simulink model "dc_motor_model_basic_blocks_current_feedback"  (Simulink 7.8)
settings: Solver=ode45  StartTime=0.0  StopTime=10.0  RelTol=1e-3
values from neighbouring files (symbols this model uses):
  I_d = 0    [dc_motor_basic_blocks_current_feedback.m]    (also in dc_motor_h_bridge_current_feedback.m)
  J = 8.85*10^(-7)    (= 8.85e-07)    [dc_motor_basic_blocks_current_feedback.m]    (also in dc_motor_h_bridge_current_feedback.m)
  k_emf = k_tau    (= 0.0452)    [dc_motor_basic_blocks_current_feedback.m]    (also in dc_motor_h_bridge_current_feedback.m)
  k_tau = 0.0452    [dc_motor_basic_blocks_current_feedback.m]    (also in dc_motor_h_bridge_current_feedback.m)
  Kd = 0    [dc_motor_basic_blocks_current_feedback.m]    (also in dc_motor_h_bridge_current_feedback.m)
  Ki = 1    [dc_motor_basic_blocks_current_feedback.m]    (also in dc_motor_h_bridge_current_feedback.m)
  Kp = 1    [dc_motor_basic_blocks_current_feedback.m]    (also in dc_motor_h_bridge_current_feedback.m)
  L = 0.746*10^(-3)    (= 0.000746)    [dc_motor_basic_blocks_current_feedback.m]    (also in dc_motor_h_bridge_current_feedback.m)
  mu = 10^(-6)    (= 1e-06)    [dc_motor_basic_blocks_current_feedback.m]    (also in dc_motor_h_bridge_current_feedback.m)
  R = 7.25    [dc_motor_basic_blocks_current_feedback.m]    (also in dc_motor_h_bridge_current_feedback.m)
  T_load = 0.1    [dc_motor_basic_blocks_current_feedback.m]    (also in dc_motor_h_bridge_current_feedback.m = 0)
  w_d = 500    [dc_motor_basic_blocks_current_feedback.m]    (also in dc_motor_h_bridge_current_feedback.m = 400)
libraries: simulink x1
settings Model: Creator=krzysztof  LastModifiedBy=krzysztof

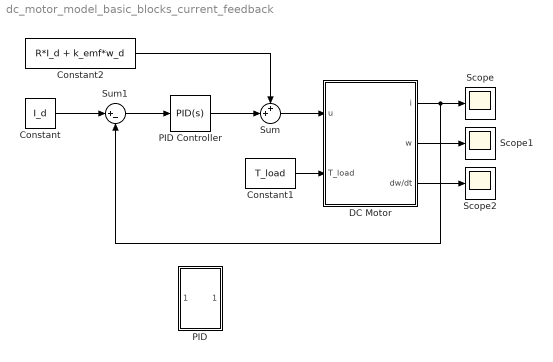
== system dc_motor_model_basic_blocks_current_feedback ==
  Constant : Constant  Value=I_d
  Constant1 : Constant  Value=T_load
  Constant2 : Constant  Value=R*I_d + k_emf*w_d
  DC Motor : Subsystem
  PID : Subsystem
  PID Controller : simulink/Continuous/PID Controller  Controller=PID  TimeDomain=Continuous-time  SampleTime=1  IntegratorMethod=Forward Euler  FilterMethod=Forward Euler  Form=Parallel  P=Kp  I=Ki  D=Kd  N=100  InitialConditionSource=internal  InitialConditionForIntegrator=0  InitialConditionForFilter=0  ExternalReset=none  LimitOutput=off  UpperSaturationLimit=inf  LowerSaturationLimit=-inf  LinearizeAsGain=off  AntiWindupMode=none  Kb=1  TrackingMode=off  Kt=1  PParamMin=[]  PParamMax=[]  IParamMin=[]  IParamMax=[]  DParamMin=[]  DParamMax=[]  NParamMin=[]  NParamMax=[]  KbParamMin=[]  KbParamMax=[]  KtParamMin=[]  KtParamMax=[]  POutMin=[]  POutMax=[]  IOutMin=[]  IOutMax=[]  DOutMin=[]  DOutMax=[]  NOutMin=[]  NOutMax=[]  KbOutMin=[]  KbOutMax=[]  KtOutMin=[]  KtOutMax=[]  IntegratorOutMin=[]  IntegratorOutMax=[]  FilterOutMin=[]  FilterOutMax=[]  SumOutMin=[]  SumOutMax=[]  SumI1OutMin=[]  SumI1OutMax=[]  SumI2OutMin=[]  SumI2OutMax=[]  SumI3OutMin=[]  SumI3OutMax=[]  SumDOutMin=[]  SumDOutMax=[]  SaturationOutMin=[]  SaturationOutMax=[]  IntegratorContinuousStateAttributes=''  IntegratorStateMustResolveToSignalObject=off  IntegratorRTWStateStorageClass=Auto  FilterContinuousStateAttributes=''  FilterStateMustResolveToSignalObject=off  FilterRTWStateStorageClass=Auto
  Scope : Scope
      settings: SaveName=i_motor
  Scope1 : Scope
      settings: SaveName=w
  Scope2 : Scope
  Sum : Sum  Inputs=++|
  Sum1 : Sum  Inputs=|+-
  wires:
  Constant1/1 -> DC Motor/2(T_load)
  DC Motor/1(i) -> Scope/1, Sum1/2
  DC Motor/3(dw/dt) -> Scope2/1
  DC Motor/2(w) -> Scope1/1
  Sum/1 -> DC Motor/1(u)
  Constant/1 -> Sum1/1
  Constant2/1 -> Sum/1
  Sum1/1 -> PID Controller/1
  PID Controller/1 -> Sum/2

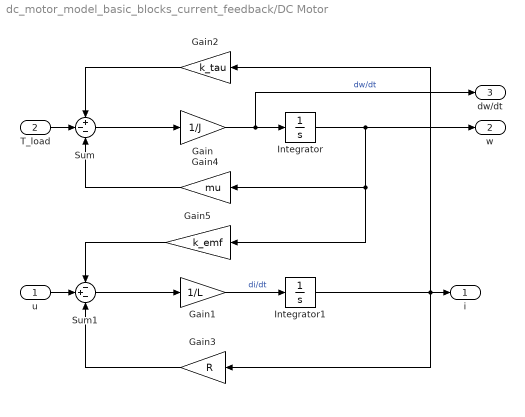
== system dc_motor_model_basic_blocks_current_feedback/DC Motor ==
  u : Inport
  T_load : Inport  Port=2
  Gain : Gain  Gain=1/J
  Gain1 : Gain  Gain=1/L
  Gain2 : Gain  Gain=k_tau
  Gain3 : Gain  Gain=R
  Gain4 : Gain  Gain=mu
  Gain5 : Gain  Gain=k_emf
  Integrator : Integrator
  Integrator1 : Integrator
  Sum : Sum  Inputs=+--
  Sum1 : Sum  Inputs=-+-
  i : Outport
  w : Outport  Port=2
  dw/dt : Outport  Port=3
  wires:
  Integrator/1 -> Gain4/1, Gain5/1, w/1
  Integrator1/1 -> Gain2/1, Gain3/1, i/1
  Gain/1 -> Integrator/1, dw/dt/1  "dw/dt"
  Gain1/1 -> Integrator1/1  "di/dt"
  Sum/1 -> Gain/1
  Sum1/1 -> Gain1/1
  Gain2/1 -> Sum/1
  Gain3/1 -> Sum1/3
  Gain4/1 -> Sum/3
  Gain5/1 -> Sum1/1
  T_load/1 -> Sum/2
  u/1 -> Sum1/2

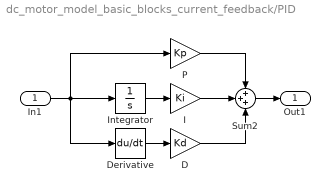
== system dc_motor_model_basic_blocks_current_feedback/PID ==
  In1 : Inport
  D : Gain  Gain=Kd
  Derivative : Derivative
  I : Gain  Gain=Ki
  Integrator : Integrator
  P : Gain  Gain=Kp
  Sum2 : Sum  Inputs=+++
  Out1 : Outport
  wires:
  Derivative/1 -> D/1
  Integrator/1 -> I/1
  P/1 -> Sum2/1
  I/1 -> Sum2/2
  D/1 -> Sum2/3
  In1/1 -> Derivative/1, Integrator/1, P/1
  Sum2/1 -> Out1/1
